simulink model "PassengerCar"  (R2019b)
settings: Solver=ode1  StartTime=0  StopTime=25  FixedStep=1.0000000000000000e-003  RelTol=1e-3
InitFcn:
  | sampleTime = str2double(get_param(bdroot, 'FixedStep'));
undefined symbols (not defined in the file or in its folder): AccPedalPos, BrakePedalPos, BrakeSwitch, DiscIntNeverNeededParam, DYNA4, EngSpd, IgnitionSwitch, InitialGear, InitialSpeed, IntendedEngTrq, LeftIndicator, MainBrakePress, MaxGear, MDL, MinGear, RefAcc, RefLane, RefLatPos, RefPath, RefPathCurv, RefSpd, RefSpdPreview, RefSpdRetrospect, RightIndicator, SteeringWheelAng, SteeringWheelTrq, UserDefinedRefValue, vm_const
libraries: UtilitiesLibrary x31, simulink x18, WheelSystemModules x13, LongitudinalControllerModules x13, LateralControllerModules x7, AnimationBusselectorModules x5, EnvironmentModules x5, BasicEngineControlModules x5, MiscellaneousControlModules x5, Animation3Modules x4, AuxiliariesModules x4, TireModules x4
(part 8 of 39)

== system PassengerCar/VehicleControl/VehicleControlOutput ==
  InitialConditions___UNIQUE_1 : Inport  Description=|
      | <name>InitialConditions</name>
      | <comment></comment>
  LongitudinalControl___UNIQUE_1 : Inport  Description=|  Port=2
      | <name>LongitudinalControl</name>
      | <comment></comment>
  LateralControl___UNIQUE_1 : Inport  Description=|  Port=3
      | <name>LateralControl</name>
      | <comment></comment>
  BrakeHydraulicsControl___UNIQUE_1 : Inport  Description=|  Port=4
      | <name>BrakeHydraulicsControl</name>
      | <comment></comment>
  EngineControl___UNIQUE_1 : Inport  Description=|  Port=5
      | <name>EngineControl</name>
      | <comment></comment>
  SuspensionTestRigControl___UNIQUE_1 : Inport  Description=|  Port=6
      | <name>SuspensionTestRigControl</name>
      | <comment></comment>
  TemperatureControl___UNIQUE_1 : Inport  Description=|  Port=7
      | <name>TemperatureControl</name>
      | <comment></comment>
  UserDefinedControl___UNIQUE_1 : Inport  Description=|  Port=8
      | <name>UserDefinedControl</name>
      | <comment></comment>
  __TDO__VehicleControl : BusCreator  Inputs=8
  VehicleControl___UNIQUE_1 : Outport  Description=|  VectorParamsAs1DForOutWhenUnconnected=off
      | <name>InitialConditions</name>
      | <comment></comment>
  wires:
  __TDO__VehicleControl/1 -> VehicleControl___UNIQUE_1/1  "VehicleControl"
  UserDefinedControl___UNIQUE_1/1 -> __TDO__VehicleControl/8  "UserDefinedControl"
  TemperatureControl___UNIQUE_1/1 -> __TDO__VehicleControl/7  "TemperatureControl"
  SuspensionTestRigControl___UNIQUE_1/1 -> __TDO__VehicleControl/6  "SuspensionTestRigControl"
  EngineControl___UNIQUE_1/1 -> __TDO__VehicleControl/5  "EngineControl"
  BrakeHydraulicsControl___UNIQUE_1/1 -> __TDO__VehicleControl/4  "BrakeHydraulicsControl"
  LateralControl___UNIQUE_1/1 -> __TDO__VehicleControl/3  "LateralControl"
  LongitudinalControl___UNIQUE_1/1 -> __TDO__VehicleControl/2  "LongitudinalControl"
  InitialConditions___UNIQUE_1/1 -> __TDO__VehicleControl/1  "InitialConditions"

== system PassengerCar/ControlUnits/ADAS/ADASOutput ==
  __SRC__ADAS.LongitudinalControlIntervention[0;1] : Constant  Value=0.0  OutDataTypeStr=Inherit: Inherit via back propagation
  __SRC__ADAS.PrioritizedADASControl.LimitsActive[0;1] : Constant  Value=0.0  OutDataTypeStr=Inherit: Inherit via back propagation
  __SRC__ADAS.PrioritizedADASControl.LowerLimitBrakePress[Pa] : Constant  Value=0.0  OutDataTypeStr=Inherit: Inherit via back propagation
  __SRC__ADAS.PrioritizedADASControl.LowerLimitTrq[Nm] : Constant  Value=-vm_const('PAR_NOT_GIVEN')  OutDataTypeStr=Inherit: Inherit via back propagation
  __SRC__ADAS.PrioritizedADASControl.UpperLimitTrq[Nm] : Constant  Value=vm_const('PAR_NOT_GIVEN')  OutDataTypeStr=Inherit: Inherit via back propagation
  __TDO__ADAS : BusCreator  Inputs=2
  __TDO__ADAS.PrioritizedADASControl : BusCreator  Inputs=4
  ADAS___UNIQUE_1 : Outport  Description=|  PortDimensions=[5]  VectorParamsAs1DForOutWhenUnconnected=off
      | <name>PrioritizedADASControl.LimitsActive[0;1]</name>
      | <comment></comment>
  wires:
  __SRC__ADAS.PrioritizedADASControl.LimitsActive[0;1]/1 -> __TDO__ADAS.PrioritizedADASControl/1  "LimitsActive[0;1]"
  __TDO__ADAS.PrioritizedADASControl/1 -> __TDO__ADAS/1  "PrioritizedADASControl"
  __SRC__ADAS.PrioritizedADASControl.UpperLimitTrq[Nm]/1 -> __TDO__ADAS.PrioritizedADASControl/2  "UpperLimitTrq[Nm]"
  __SRC__ADAS.PrioritizedADASControl.LowerLimitTrq[Nm]/1 -> __TDO__ADAS.PrioritizedADASControl/3  "LowerLimitTrq[Nm]"
  __SRC__ADAS.PrioritizedADASControl.LowerLimitBrakePress[Pa]/1 -> __TDO__ADAS.PrioritizedADASControl/4  "LowerLimitBrakePress[Pa]"
  __SRC__ADAS.LongitudinalControlIntervention[0;1]/1 -> __TDO__ADAS/2  "LongitudinalControlIntervention[0;1]"
  __TDO__ADAS/1 -> ADAS___UNIQUE_1/1  "ADAS"

== system PassengerCar/ControlUnits/ADAS/DynaComponentInfo ==

== system PassengerCar/ControlUnits/LCU/DynaComponentInfo ==

== system PassengerCar/ControlUnits/LCU/LCUOutput ==
  VehicleLights___UNIQUE_1 : Inport  Description=|
      | <name>VehicleLights</name>
      | <comment></comment>
  __TDO__LCU : BusCreator  Inputs=1
  LCU___UNIQUE_1 : Outport  Description=|  VectorParamsAs1DForOutWhenUnconnected=off
      | <name>VehicleLights</name>
      | <comment></comment>
  wires:
  VehicleLights___UNIQUE_1/1 -> __TDO__LCU/1  "VehicleLights"
  __TDO__LCU/1 -> LCU___UNIQUE_1/1  "LCU"

== system PassengerCar/ControlUnits/StateSensors/DynaComponentInfo ==

== system PassengerCar/ControlUnits/StateSensors/StateSensorsOutput ==
  IMU___UNIQUE_1 : Inport  Description=|
      | <name>IMU</name>
      | <comment></comment>
  __TDO__StateSensors : BusCreator  Inputs=1
  StateSensors___UNIQUE_1 : Outport  Description=|  VectorParamsAs1DForOutWhenUnconnected=off
      | <name>IMU</name>
      | <comment></comment>
  wires:
  IMU___UNIQUE_1/1 -> __TDO__StateSensors/1  "IMU"
  __TDO__StateSensors/1 -> StateSensors___UNIQUE_1/1  "StateSensors"

== system PassengerCar/ControlUnits/VCU/DynaComponentInfo ==

== system PassengerCar/ControlUnits/VCU/InputFromADAS ==
  fromADAS : Inport  Description=|
      | <name>DriverBrakePedalMode[0;1;2]</name>
      | <comment></comment>
  TDBusSelector : BusSelector  OutputSignals=PrioritizedADASControl
  __TDO__PrioritizedADASControl : BusCreator  Inputs=1
  PrioritizedADASControl___UNIQUE_1 : Outport  Description=|
      | <name>PrioritizedADASControl</name>
      | <comment></comment>
  wires:
  fromADAS/1 -> TDBusSelector/1  "ControlSignals"
  TDBusSelector/1 -> __TDO__PrioritizedADASControl/1  "<PrioritizedADASControl>"
  __TDO__PrioritizedADASControl/1 -> PrioritizedADASControl___UNIQUE_1/1  "PrioritizedADASControl"

== system PassengerCar/ControlUnits/VCU/InputFromCTRL ==
  fromCTRL : Inport
  TDBusSelector : BusSelector  OutputSignals=CTRL.LongitudinalControl.AccPedalPos[0_1],CTRL.LongitudinalControl.BrakePedalPos[0_1],CTRL.LongitudinalControl.DriverInfo.MeanEngMaxTrq[Nm],CTRL.LongitudinalControl.DriverInfo.MeanEngDragTrq[Nm],CTRL.LongitudinalControl.DriverInfo.ThirtyPercentAccPedalEngTrq[Nm]
  __TDD__AccPedalPos[0_1] : Demux  Outputs=[1]
  __TDD__BrakePedalPos[0_1] : Demux  Outputs=1
  __TDD__MeanEngDragTrq[Nm] : Demux  Outputs=[1]
  __TDD__MeanEngMaxTrq[Nm] : Demux  Outputs=[1]
  __TDD__ThirtyPercentAccPedalEngTrq[Nm] : Demux  Outputs=[1]
  AccPedalPos[0_1] : Outport  Description=|  PortDimensions=[1]  VectorParamsAs1DForOutWhenUnconnected=off
      | <name>CTRL.LongitudinalControl.AccPedalPos[0_1]</name>
      | <comment>Accelerator pedal position</comment>
  BrakePedalPos[0_1]___UNIQUE_1 : Outport  Description=|  Port=2  VectorParamsAs1DForOutWhenUnconnected=off
      | <name>CTRL.LongitudinalControl.BrakePedalPos[0_1]</name>
      | <comment></comment>
  MeanEngMaxTrq[Nm]___UNIQUE_1 : Outport  Description=|  Port=3  PortDimensions=[1]  VectorParamsAs1DForOutWhenUnconnected=off
      | <name>CTRL.LongitudinalControl.DriverInfo.MeanEngMaxTrq[Nm]</name>
      | <comment></comment>
  MeanEngDragTrq[Nm]___UNIQUE_1 : Outport  Description=|  Port=4  PortDimensions=[1]  VectorParamsAs1DForOutWhenUnconnected=off
      | <name>CTRL.LongitudinalControl.DriverInfo.MeanEngDragTrq[Nm]</name>
      | <comment></comment>
  ThirtyPercentAccPedalEngTrq[Nm]___UNIQUE_1 : Outport  Description=|  Port=5  PortDimensions=[1]
      | <name>CTRL.LongitudinalControl.DriverInfo.ThirtyPercentAccPedalEngTrq[Nm]</name>
      | <comment></comment>
  wires:
  __TDD__ThirtyPercentAccPedalEngTrq[Nm]/1 -> ThirtyPercentAccPedalEngTrq[Nm]___UNIQUE_1/1  "ThirtyPercentAccPedalEngTrq[Nm]"
  __TDD__MeanEngDragTrq[Nm]/1 -> MeanEngDragTrq[Nm]___UNIQUE_1/1  "MeanEngDragTrq[Nm]"
  __TDD__MeanEngMaxTrq[Nm]/1 -> MeanEngMaxTrq[Nm]___UNIQUE_1/1  "MeanEngMaxTrq[Nm]"
  __TDD__BrakePedalPos[0_1]/1 -> BrakePedalPos[0_1]___UNIQUE_1/1  "BrakePedalPos[0_1]"
  __TDD__AccPedalPos[0_1]/1 -> AccPedalPos[0_1]/1  "AccPedalPos[0_1]"
  TDBusSelector/5 -> __TDD__ThirtyPercentAccPedalEngTrq[Nm]/1  "<ThirtyPercentAccPedalEngTrq[Nm]>"
  TDBusSelector/4 -> __TDD__MeanEngDragTrq[Nm]/1  "<MeanEngDragTrq[Nm]>"
  TDBusSelector/3 -> __TDD__MeanEngMaxTrq[Nm]/1  "<MeanEngMaxTrq[Nm]>"
  TDBusSelector/2 -> __TDD__BrakePedalPos[0_1]/1  "<BrakePedalPos[0_1]>"
  TDBusSelector/1 -> __TDD__AccPedalPos[0_1]/1  "<AccPedalPos[0_1]>"
  fromCTRL/1 -> TDBusSelector/1

== system PassengerCar/ControlUnits/VCU/InputFromVehicle ==
  fromVehicle : Inport
  TDBusSelector : BusSelector  OutputSignals=BrakeSystem.BrakeSystemPhysics.MaxMainBrakePress[Pa]
  __TDD__MaxMainBrakePress[Pa] : Demux  Outputs=[1]
  MaxMainBrakePress[Pa]___UNIQUE_1 : Outport  Description=|  PortDimensions=[1]  VectorParamsAs1DForOutWhenUnconnected=off
      | <name>BrakeSystem.BrakeSystemPhysics.MaxMainBrakePress[Pa]</name>
      | <comment>Maximum main brake pressure</comment>
  wires:
  fromVehicle/1 -> TDBusSelector/1
  TDBusSelector/1 -> __TDD__MaxMainBrakePress[Pa]/1  "<MaxMainBrakePress[Pa]>"
  __TDD__MaxMainBrakePress[Pa]/1 -> MaxMainBrakePress[Pa]___UNIQUE_1/1  "MaxMainBrakePress[Pa]"

== system PassengerCar/ControlUnits/VCU/VCUOutput ==
  TransmissionLoad[0_1]___UNIQUE_1 : Inport  Description=|  PortDimensions=[1]
      | <name>TransmissionLoad[0_1]</name>
      | <comment></comment>
  IntendedEngTrq[Nm]___UNIQUE_1 : Inport  Description=|  Port=2  PortDimensions=[1]
      | <name>IntendedEngTrq[Nm]</name>
      | <comment>Intended torque of engine</comment>
  IntendedEngTrqActive[0;1]___UNIQUE_1 : Inport  Description=|  Port=3  PortDimensions=[1]
      | <name>IntendedEngTrqActive[0;1]</name>
      | <comment></comment>
  IntendedMainBrakePress[Pa]___UNIQUE_1 : Inport  Description=|  Port=4  PortDimensions=[1]
      | <name>IntendedMainBrakePress[Pa]</name>
      | <comment></comment>
  IntendedMainBrakePressActive[0;1]___UNIQUE_1 : Inport  Description=|  Port=5  PortDimensions=[1]
      | <name>IntendedMainBrakePressActive[0;1]</name>
      | <comment></comment>
  __SAT__VCU.EngRunPermission[0;1] : Saturate  UpperLimit=1  LowerLimit=0
  __SRC__VCU.DriverInfo.ConventionalVehicleSwitch[0;1] : Constant  Value=1.0  OutDataTypeStr=Inherit: Inherit via back propagation
  __SRC__VCU.DrivingState[-] : Constant  Value=0.0  OutDataTypeStr=Inherit: Inherit via back propagation
  __SRC__VCU.EngRunPermission[0;1] : Constant  Value=1.0  OutDataTypeStr=Inherit: Inherit via back propagation
  __TDD__VCU.IntendedEngTrqActive[0;1] : Demux  Outputs=[1]
  __TDD__VCU.IntendedEngTrq[Nm] : Demux  Outputs=[1]
  __TDD__VCU.IntendedMainBrakePressActive[0;1] : Demux  Outputs=[1]
  __TDD__VCU.IntendedMainBrakePress[Pa] : Demux  Outputs=[1]
  __TDD__VCU.TransmissionLoad[0_1] : Demux  Outputs=[1]
  __TDO__VCU : BusCreator  Inputs=8
  __TDO__VCU.DriverInfo : BusCreator  Inputs=1
  VCU___UNIQUE_1 : Outport  Description=|  PortDimensions=[8]  VectorParamsAs1DForOutWhenUnconnected=off
      | <name>TransmissionLoad[0_1]</name>
      | <comment></comment>
  wires:
  __SRC__VCU.EngRunPermission[0;1]/1 -> __SAT__VCU.EngRunPermission[0;1]/1
  TransmissionLoad[0_1]___UNIQUE_1/1 -> __TDD__VCU.TransmissionLoad[0_1]/1
  __TDD__VCU.TransmissionLoad[0_1]/1 -> __TDO__VCU/1  "TransmissionLoad[0_1]"
  IntendedEngTrq[Nm]___UNIQUE_1/1 -> __TDD__VCU.IntendedEngTrq[Nm]/1
  __TDD__VCU.IntendedEngTrq[Nm]/1 -> __TDO__VCU/2  "IntendedEngTrq[Nm]"
  IntendedEngTrqActive[0;1]___UNIQUE_1/1 -> __TDD__VCU.IntendedEngTrqActive[0;1]/1
  __TDD__VCU.IntendedEngTrqActive[0;1]/1 -> __TDO__VCU/3  "IntendedEngTrqActive[0;1]"
  IntendedMainBrakePress[Pa]___UNIQUE_1/1 -> __TDD__VCU.IntendedMainBrakePress[Pa]/1
  __TDD__VCU.IntendedMainBrakePress[Pa]/1 -> __TDO__VCU/4  "IntendedMainBrakePress[Pa]"
  IntendedMainBrakePressActive[0;1]___UNIQUE_1/1 -> __TDD__VCU.IntendedMainBrakePressActive[0;1]/1
  __TDD__VCU.IntendedMainBrakePressActive[0;1]/1 -> __TDO__VCU/5  "IntendedMainBrakePressActive[0;1]"
  __SRC__VCU.DrivingState[-]/1 -> __TDO__VCU/6  "DrivingState[-]"
  __SRC__VCU.DriverInfo.ConventionalVehicleSwitch[0;1]/1 -> __TDO__VCU.DriverInfo/1  "ConventionalVehicleSwitch[0;1]"
  __TDO__VCU.DriverInfo/1 -> __TDO__VCU/7  "DriverInfo"
  __SAT__VCU.EngRunPermission[0;1]/1 -> __TDO__VCU/8  "EngRunPermission[0;1]"
  __TDO__VCU/1 -> VCU___UNIQUE_1/1  "VCU"

== system PassengerCar/Environment/Road/DynaSystemInfo ==

== system PassengerCar/Traffic/TrafficOutputs/DistanceToVehicleOutput ==
  LeftAdjacentLaneFrontalDist[m]___UNIQUE_1 : Inport  Description=|  PortDimensions=[1]
      | <name>LeftAdjacentLaneFrontalDist[m]</name>
      | <comment>Distance of VuT to next frontal traffic object on left adjacent lane</comment>
  LeftAdjacentLaneRearDist[m]___UNIQUE_1 : Inport  Description=|  Port=2  PortDimensions=[1]
      | <name>LeftAdjacentLaneRearDist[m]</name>
      | <comment>Distance of VuT to next rear traffic object on left adjacent lane</comment>
  MyLaneFrontalDist[m]___UNIQUE_1 : Inport  Description=|  Port=3  PortDimensions=[1]
      | <name>MyLaneFrontalDist[m]</name>
      | <comment>Distance of VuT to next frontal traffic object on the same lane</comment>
  MyLaneRearDist[m]___UNIQUE_1 : Inport  Description=|  Port=4  PortDimensions=[1]
      | <name>MyLaneRearDist[m]</name>
      | <comment>Distance of VuT to next rear traffic object on the same lane</comment>
  RightAdjacentLaneFrontalDist[m]___UNIQUE_1 : Inport  Description=|  Port=5  PortDimensions=[1]
      | <name>RightAdjacentLaneFrontalDist[m]</name>
      | <comment>Distance of VuT to next frontal traffic object on right adjacent lane</comment>
  RightAdjacentLaneRearDist[m]___UNIQUE_1 : Inport  Description=|  Port=6  PortDimensions=[1]
      | <name>RightAdjacentLaneRearDist[m]</name>
      | <comment>Distance of VuT to next rear traffic object on right adjacent lane</comment>
  LeftAdjacentLaneFrontalSpd[m/s]___UNIQUE_1 : Inport  Description=|  Port=7  PortDimensions=[1]
      | <name>LeftAdjacentLaneFrontalSpd[m/s]</name>
      | <comment>Longitudinal speed of next frontal traffic object on left adjacent lane</comment>
  LeftAdjacentLaneRearSpd[m/s]___UNIQUE_1 : Inport  Description=|  Port=8  PortDimensions=[1]
      | <name>LeftAdjacentLaneRearSpd[m/s]</name>
      | <comment>Longitudinal speed of next rear traffic object on left adjacent lane</comment>
  MyLaneFrontalSpd[m/s]___UNIQUE_1 : Inport  Description=|  Port=9  PortDimensions=[1]
      | <name>MyLaneFrontalSpd[m/s]</name>
      | <comment>Longitudinal speed of next frontal traffic object on the same lane</comment>
  MyLaneRearSpd[m/s]___UNIQUE_1 : Inport  Description=|  Port=10  PortDimensions=[1]
      | <name>MyLaneRearSpd[m/s]</name>
      | <comment>Longitudinal speed of next rear traffic object on the same lane</comment>
  RightAdjacentLaneFrontalSpd[m/s]___UNIQUE_1 : Inport  Description=|  Port=11  PortDimensions=[1]
      | <name>RightAdjacentLaneFrontalSpd[m/s]</name>
      | <comment>Longitudinal speed of next frontal traffic object on right adjacent lane</comment>
  RightAdjacentLaneRearSpd[m/s]___UNIQUE_1 : Inport  Description=|  Port=12  PortDimensions=[1]
      | <name>RightAdjacentLaneRearSpd[m/s]</name>
      | <comment>Longitudinal speed of next rear traffic object on right adjacent lane</comment>
  __TDD__Traffic.AdjacentObjectsSpeeds.LeftAdjacentLaneFrontalSpd[m/s] : Demux  Outputs=[1]
  __TDD__Traffic.AdjacentObjectsSpeeds.LeftAdjacentLaneRearSpd[m/s] : Demux  Outputs=[1]
  __TDD__Traffic.AdjacentObjectsSpeeds.MyLaneFrontalSpd[m/s] : Demux  Outputs=[1]
  __TDD__Traffic.AdjacentObjectsSpeeds.MyLaneRearSpd[m/s] : Demux  Outputs=[1]
  __TDD__Traffic.AdjacentObjectsSpeeds.RightAdjacentLaneFrontalSpd[m/s] : Demux  Outputs=[1]
  __TDD__Traffic.AdjacentObjectsSpeeds.RightAdjacentLaneRearSpd[m/s] : Demux  Outputs=[1]
  __TDD__Traffic.DistancesToVehicle.LeftAdjacentLaneFrontalDist[m] : Demux  Outputs=[1]
  __TDD__Traffic.DistancesToVehicle.LeftAdjacentLaneRearDist[m] : Demux  Outputs=[1]
  __TDD__Traffic.DistancesToVehicle.MyLaneFrontalDist[m] : Demux  Outputs=[1]
  __TDD__Traffic.DistancesToVehicle.MyLaneRearDist[m] : Demux  Outputs=[1]
  __TDD__Traffic.DistancesToVehicle.RightAdjacentLaneFrontalDist[m] : Demux  Outputs=[1]
  __TDD__Traffic.DistancesToVehicle.RightAdjacentLaneRearDist[m] : Demux  Outputs=[1]
  __TDO__Traffic : BusCreator  Inputs=2
  __TDO__Traffic.AdjacentObjectsSpeeds : BusCreator  Inputs=6
  __TDO__Traffic.DistancesToVehicle : BusCreator  Inputs=6
  Traffic___UNIQUE_1 : Outport  Description=|  PortDimensions=[12]  VectorParamsAs1DForOutWhenUnconnected=off
      | <name>LeftAdjacentLaneFrontalDist[m]</name>
      | <comment>Distance of VuT to next frontal traffic object on left adjacent lane</comment>
  wires:
  LeftAdjacentLaneFrontalDist[m]___UNIQUE_1/1 -> __TDD__Traffic.DistancesToVehicle.LeftAdjacentLaneFrontalDist[m]/1
  __TDD__Traffic.DistancesToVehicle.LeftAdjacentLaneFrontalDist[m]/1 -> __TDO__Traffic.DistancesToVehicle/1  "LeftAdjacentLaneFrontalDist[m]"
  __TDO__Traffic.DistancesToVehicle/1 -> __TDO__Traffic/1  "DistancesToVehicle"
  LeftAdjacentLaneRearDist[m]___UNIQUE_1/1 -> __TDD__Traffic.DistancesToVehicle.LeftAdjacentLaneRearDist[m]/1
  __TDD__Traffic.DistancesToVehicle.LeftAdjacentLaneRearDist[m]/1 -> __TDO__Traffic.DistancesToVehicle/2  "LeftAdjacentLaneRearDist[m]"
  MyLaneFrontalDist[m]___UNIQUE_1/1 -> __TDD__Traffic.DistancesToVehicle.MyLaneFrontalDist[m]/1
  __TDD__Traffic.DistancesToVehicle.MyLaneFrontalDist[m]/1 -> __TDO__Traffic.DistancesToVehicle/3  "MyLaneFrontalDist[m]"
  MyLaneRearDist[m]___UNIQUE_1/1 -> __TDD__Traffic.DistancesToVehicle.MyLaneRearDist[m]/1
  __TDD__Traffic.DistancesToVehicle.MyLaneRearDist[m]/1 -> __TDO__Traffic.DistancesToVehicle/4  "MyLaneRearDist[m]"
  RightAdjacentLaneFrontalDist[m]___UNIQUE_1/1 -> __TDD__Traffic.DistancesToVehicle.RightAdjacentLaneFrontalDist[m]/1
  __TDD__Traffic.DistancesToVehicle.RightAdjacentLaneFrontalDist[m]/1 -> __TDO__Traffic.DistancesToVehicle/5  "RightAdjacentLaneFrontalDist[m]"
  RightAdjacentLaneRearDist[m]___UNIQUE_1/1 -> __TDD__Traffic.DistancesToVehicle.RightAdjacentLaneRearDist[m]/1
  __TDD__Traffic.DistancesToVehicle.RightAdjacentLaneRearDist[m]/1 -> __TDO__Traffic.DistancesToVehicle/6  "RightAdjacentLaneRearDist[m]"
  LeftAdjacentLaneFrontalSpd[m/s]___UNIQUE_1/1 -> __TDD__Traffic.AdjacentObjectsSpeeds.LeftAdjacentLaneFrontalSpd[m/s]/1
  __TDD__Traffic.AdjacentObjectsSpeeds.LeftAdjacentLaneFrontalSpd[m/s]/1 -> __TDO__Traffic.AdjacentObjectsSpeeds/1  "LeftAdjacentLaneFrontalSpd[m/s]"
  __TDO__Traffic.AdjacentObjectsSpeeds/1 -> __TDO__Traffic/2  "AdjacentObjectsSpeeds"
  LeftAdjacentLaneRearSpd[m/s]___UNIQUE_1/1 -> __TDD__Traffic.AdjacentObjectsSpeeds.LeftAdjacentLaneRearSpd[m/s]/1
  __TDD__Traffic.AdjacentObjectsSpeeds.LeftAdjacentLaneRearSpd[m/s]/1 -> __TDO__Traffic.AdjacentObjectsSpeeds/2  "LeftAdjacentLaneRearSpd[m/s]"
  MyLaneFrontalSpd[m/s]___UNIQUE_1/1 -> __TDD__Traffic.AdjacentObjectsSpeeds.MyLaneFrontalSpd[m/s]/1
  __TDD__Traffic.AdjacentObjectsSpeeds.MyLaneFrontalSpd[m/s]/1 -> __TDO__Traffic.AdjacentObjectsSpeeds/3  "MyLaneFrontalSpd[m/s]"
  MyLaneRearSpd[m/s]___UNIQUE_1/1 -> __TDD__Traffic.AdjacentObjectsSpeeds.MyLaneRearSpd[m/s]/1
  __TDD__Traffic.AdjacentObjectsSpeeds.MyLaneRearSpd[m/s]/1 -> __TDO__Traffic.AdjacentObjectsSpeeds/4  "MyLaneRearSpd[m/s]"
  RightAdjacentLaneFrontalSpd[m/s]___UNIQUE_1/1 -> __TDD__Traffic.AdjacentObjectsSpeeds.RightAdjacentLaneFrontalSpd[m/s]/1
  __TDD__Traffic.AdjacentObjectsSpeeds.RightAdjacentLaneFrontalSpd[m/s]/1 -> __TDO__Traffic.AdjacentObjectsSpeeds/5  "RightAdjacentLaneFrontalSpd[m/s]"
  RightAdjacentLaneRearSpd[m/s]___UNIQUE_1/1 -> __TDD__Traffic.AdjacentObjectsSpeeds.RightAdjacentLaneRearSpd[m/s]/1
  __TDD__Traffic.AdjacentObjectsSpeeds.RightAdjacentLaneRearSpd[m/s]/1 -> __TDO__Traffic.AdjacentObjectsSpeeds/6  "RightAdjacentLaneRearSpd[m/s]"
  __TDO__Traffic/1 -> Traffic___UNIQUE_1/1  "Traffic"

== system PassengerCar/Vehicle/Auxiliaries/AuxiliariesOutput ==
  GeneratorCurr[A]___UNIQUE_1 : Inport  Description=|  PortDimensions=[1]
      | <name>GeneratorCurr[A]</name>
      | <comment></comment>
  GeneratorTrq[Nm]___UNIQUE_1 : Inport  Description=|  Port=2  PortDimensions=[1]
      | <name>GeneratorTrq[Nm]</name>
      | <comment></comment>
  GeneratorInrt[kgm^2]___UNIQUE_1 : Inport  Description=|  Port=3  PortDimensions=[1]
      | <name>GeneratorInrt[kgm^2]</name>
      | <comment></comment>
  StarterCurr[A]___UNIQUE_1 : Inport  Description=|  Port=4  PortDimensions=[1]
      | <name>StarterCurr[A]</name>
      | <comment></comment>
  StarterTrq[Nm]___UNIQUE_1 : Inport  Description=|  Port=5  PortDimensions=[1]
      | <name>StarterTrq[Nm]</name>
      | <comment></comment>
  StarterInrt[kgm**2]___UNIQUE_1 : Inport  Description=|  Port=6  PortDimensions=[1]
      | <name>StarterInrt[kgm**2]</name>
      | <comment></comment>
  __TDD__Auxiliaries.GeneratorCurr[A] : Demux  Outputs=[1]
  __TDD__Auxiliaries.GeneratorInrt[kgm^2] : Demux  Outputs=[1]
  __TDD__Auxiliaries.GeneratorTrq[Nm] : Demux  Outputs=[1]
  __TDD__Auxiliaries.StarterCurr[A] : Demux  Outputs=[1]
  __TDD__Auxiliaries.StarterInrt[kgm**2] : Demux  Outputs=[1]
  __TDD__Auxiliaries.StarterTrq[Nm] : Demux  Outputs=[1]
  __TDO__Auxiliaries : BusCreator  Inputs=6
  Auxiliaries___UNIQUE_1 : Outport  Description=|  PortDimensions=[6]  VectorParamsAs1DForOutWhenUnconnected=off
      | <name>GeneratorCurr[A]</name>
      | <comment></comment>
  wires:
  __TDO__Auxiliaries/1 -> Auxiliaries___UNIQUE_1/1  "Auxiliaries"
  __TDD__Auxiliaries.StarterInrt[kgm**2]/1 -> __TDO__Auxiliaries/6  "StarterInrt[kgm**2]"
  StarterInrt[kgm**2]___UNIQUE_1/1 -> __TDD__Auxiliaries.StarterInrt[kgm**2]/1
  __TDD__Auxiliaries.StarterTrq[Nm]/1 -> __TDO__Auxiliaries/5  "StarterTrq[Nm]"
  StarterTrq[Nm]___UNIQUE_1/1 -> __TDD__Auxiliaries.StarterTrq[Nm]/1
  __TDD__Auxiliaries.StarterCurr[A]/1 -> __TDO__Auxiliaries/4  "StarterCurr[A]"
  StarterCurr[A]___UNIQUE_1/1 -> __TDD__Auxiliaries.StarterCurr[A]/1
  __TDD__Auxiliaries.GeneratorInrt[kgm^2]/1 -> __TDO__Auxiliaries/3  "GeneratorInrt[kgm^2]"
  GeneratorInrt[kgm^2]___UNIQUE_1/1 -> __TDD__Auxiliaries.GeneratorInrt[kgm^2]/1
  __TDD__Auxiliaries.GeneratorTrq[Nm]/1 -> __TDO__Auxiliaries/2  "GeneratorTrq[Nm]"
  GeneratorTrq[Nm]___UNIQUE_1/1 -> __TDD__Auxiliaries.GeneratorTrq[Nm]/1
  __TDD__Auxiliaries.GeneratorCurr[A]/1 -> __TDO__Auxiliaries/1  "GeneratorCurr[A]"
  GeneratorCurr[A]___UNIQUE_1/1 -> __TDD__Auxiliaries.GeneratorCurr[A]/1

== system PassengerCar/Vehicle/Auxiliaries/DynaComponentInfo ==

== system PassengerCar/Vehicle/Auxiliaries/Generator ==
  EngSpd [rad/s] : Inport
  GeneratorVoltage [V] : Inport  Port=2
  RefVoltage [V] : Inport  Port=3
  LRTime [s] : Inport  Port=4
  Temp [K] : Inport  Port=5
  BattVoltage [V] : Inport  Port=6
  Alternator : AuxiliariesModules/Alternator  DATA_NODE=MDL.Vehicle.Auxiliaries.Alternator  trq_table=MDL.Vehicle.Auxiliaries.Alternator.TrqMap  max_current=MDL.Vehicle.Auxiliaries.Alternator.MaxCurrMap  max_current_rate=MDL.Vehicle.Auxiliaries.Alternator.MaxCurrRate  ref_volt=MDL.Vehicle.Auxiliaries.Alternator.RefVoltage  resist=MDL.Vehicle.Auxiliaries.Alternator.Resist  ratio=MDL.Vehicle.Auxiliaries.Alternator.SpdRatio  Inrt=MDL.Vehicle.Auxiliaries.Alternator.Inrt
  InitCurr [A] : Constant  Value=0
  VoltageRegulator : AuxiliariesModules/VoltageRegulator  DATA_NODE=MDL.Vehicle.Auxiliaries.VoltageRegulator  min_lr=MDL.Vehicle.Auxiliaries.VoltageRegulator.MinLoadResponseTime  LR_thres=MDL.Vehicle.Auxiliaries.VoltageRegulator.LoadResponseSpdLimit
  Curr [A] : Outport  VectorParamsAs1DForOutWhenUnconnected=off
  Trq [Nm] : Outport  Port=2  VectorParamsAs1DForOutWhenUnconnected=off
  Inrt [kgm**2] : Outport  Port=3  VectorParamsAs1DForOutWhenUnconnected=off
  wires:
  VoltageRegulator/1 -> Alternator/1
  EngSpd [rad/s]/1 -> VoltageRegulator/1, Alternator/2
  GeneratorVoltage [V]/1 -> Alternator/3
  InitCurr [A]/1 -> VoltageRegulator/5
  Alternator/4 -> VoltageRegulator/6
  RefVoltage [V]/1 -> VoltageRegulator/3
  LRTime [s]/1 -> VoltageRegulator/4
  Alternator/1 -> Curr [A]/1
  Alternator/2 -> Trq [Nm]/1
  Alternator/3 -> Inrt [kgm**2]/1
  Temp [K]/1 -> Alternator/4
  BattVoltage [V]/1 -> VoltageRegulator/2

== system PassengerCar/Vehicle/Auxiliaries/InputFromCTRL ==
  fromCTRL : Inport
  TDBusSelector : BusSelector  OutputSignals=CTRL.LongitudinalControl.StarterSwitch[0;1],CTRL.EnvironmentalConditions.AmbTemp[K]
  __TDD__AmbTemp[K] : Demux  Outputs=[1]
  __TDD__StarterSwitch[0;1] : Demux  Outputs=[1]
  StarterSwitch[0;1]___UNIQUE_1 : Outport  Description=|  PortDimensions=[1]  VectorParamsAs1DForOutWhenUnconnected=off
      | <name>CTRL.LongitudinalControl.StarterSwitch[0;1]</name>
      | <comment>Engine starter switch</comment>
  AmbTemp[K]___UNIQUE_1 : Outport  Description=|  Port=2  PortDimensions=[1]  VectorParamsAs1DForOutWhenUnconnected=off
      | <name>CTRL.EnvironmentalConditions.AmbTemp[K]</name>
      | <comment></comment>
  wires:
  __TDD__AmbTemp[K]/1 -> AmbTemp[K]___UNIQUE_1/1  "AmbTemp[K]"
  __TDD__StarterSwitch[0;1]/1 -> StarterSwitch[0;1]___UNIQUE_1/1  "StarterSwitch[0;1]"
  TDBusSelector/2 -> __TDD__AmbTemp[K]/1  "<AmbTemp[K]>"
  TDBusSelector/1 -> __TDD__StarterSwitch[0;1]/1  "<StarterSwitch[0;1]>"
  fromCTRL/1 -> TDBusSelector/1

== system PassengerCar/Vehicle/Auxiliaries/InputFromDrivetrain ==
  fromDrivetrain : Inport
  TDBusSelector : BusSelector  OutputSignals=DrivetrainPhysics.EngSpd[rad/s]
  __TDD__EngSpd[rad/s] : Demux  Outputs=1
  EngSpd[rad/s] : Outport  Description=|  VectorParamsAs1DForOutWhenUnconnected=off
      | <name>DrivetrainPhysics.EngSpd[rad/s]</name>
      | <comment></comment>
  wires:
  __TDD__EngSpd[rad/s]/1 -> EngSpd[rad/s]/1  "EngSpd[rad/s]"
  TDBusSelector/1 -> __TDD__EngSpd[rad/s]/1  "<EngSpd[rad/s]>"
  fromDrivetrain/1 -> TDBusSelector/1

== system PassengerCar/Vehicle/Auxiliaries/InputFromElectricalSystem ==
  fromPowernet : Inport
  TDBusSelector : BusSelector  OutputSignals=GeneratorVoltage[V],LowVoltageBattery.LowVoltageBatteryVoltage[V],StarterVoltage[V]
  __TDD__GeneratorVoltage[V] : Demux  Outputs=[1]
  __TDD__LowVoltageBatteryVoltage[V] : Demux  Outputs=[1]
  __TDD__StarterVoltage[V] : Demux  Outputs=[1]
  GeneratorVoltage[V]___UNIQUE_1 : Outport  Description=|  PortDimensions=[1]  VectorParamsAs1DForOutWhenUnconnected=off
      | <name>GeneratorVoltage[V]</name>
      | <comment></comment>
  LowVoltageBatteryVoltage[V]___UNIQUE_1 : Outport  Description=|  Port=2  PortDimensions=[1]  VectorParamsAs1DForOutWhenUnconnected=off
      | <name>LowVoltageBattery.LowVoltageBatteryVoltage[V]</name>
      | <comment></comment>
  StarterVoltage[V]___UNIQUE_1 : Outport  Description=|  Port=3  PortDimensions=[1]  VectorParamsAs1DForOutWhenUnconnected=off
      | <name>StarterVoltage[V]</name>
      | <comment></comment>
  wires:
  __TDD__StarterVoltage[V]/1 -> StarterVoltage[V]___UNIQUE_1/1  "StarterVoltage[V]"
  __TDD__LowVoltageBatteryVoltage[V]/1 -> LowVoltageBatteryVoltage[V]___UNIQUE_1/1  "LowVoltageBatteryVoltage[V]"
  __TDD__GeneratorVoltage[V]/1 -> GeneratorVoltage[V]___UNIQUE_1/1  "GeneratorVoltage[V]"
  TDBusSelector/3 -> __TDD__StarterVoltage[V]/1  "<StarterVoltage[V]>"
  TDBusSelector/2 -> __TDD__LowVoltageBatteryVoltage[V]/1  "<LowVoltageBatteryVoltage[V]>"
  TDBusSelector/1 -> __TDD__GeneratorVoltage[V]/1  "<GeneratorVoltage[V]>"
  fromPowernet/1 -> TDBusSelector/1

== system PassengerCar/Vehicle/Auxiliaries/SimpleEnergyManagement ==
  StarterSwitch [0;1] : Inport
  Generator off : Constant  Value=0
  GeneratorReferenceVoltage : LookupTableModules/ConstantVoltage  DATA_NODE=MDL.Vehicle.Auxiliaries.GeneratorReferenceVoltage  ConstVoltage=MDL.Vehicle.Auxiliaries.GeneratorReferenceVoltage.Voltage
  Switch : Switch  Threshold=0.5
  RefVoltage [V] : Outport  VectorParamsAs1DForOutWhenUnconnected=off
  wires:
  GeneratorReferenceVoltage/1 -> Switch/3
  Switch/1 -> RefVoltage [V]/1
  StarterSwitch [0;1]/1 -> Switch/2
  Generator off/1 -> Switch/1

== system PassengerCar/Vehicle/Auxiliaries/Starter ==
  StarterVoltage [V] : Inport
  EngSpd [rad/s] : Inport  Port=2
  StarterSwitch [0;1] : Inport  Port=3
  Temp [K] : Inport  Port=4
  PermanentMagnetDCMotor : AuxiliariesModules/PermanentMagnetDCMotor  DATA_NODE=MDL.Vehicle.Auxiliaries.PermanentMagnetDCMotor  flux=MDL.Vehicle.Auxiliaries.PermanentMagnetDCMotor.FieldFlux  armature_inductance=MDL.Vehicle.Auxiliaries.PermanentMagnetDCMotor.ArmatureInduct  armature_resistance=MDL.Vehicle.Auxiliaries.PermanentMagnetDCMotor.ArmatureResistCurve  motor_const=MDL.Vehicle.Auxiliaries.PermanentMagnetDCMotor.MotorConst  inrt=MDL.Vehicle.Auxiliaries.PermanentMagnetDCMotor.Inrt  heat_cap=MDL.Vehicle.Auxiliaries.PermanentMagnetDCMotor.HeatCap
  StarterControl : AuxiliariesModules/StarterControl  DATA_NODE=MDL.Vehicle.Auxiliaries.StarterControl  speedratio=MDL.Vehicle.Auxiliaries.StarterControl.StarterEngSpdRatio
  Terminator : Terminator
  Terminator1 : Terminator
  Terminator2 : Terminator
  StarterCurr [A] : Outport  VectorParamsAs1DForOutWhenUnconnected=off
  StarterTrq [Nm] : Outport  Port=2  VectorParamsAs1DForOutWhenUnconnected=off
  StarterInrt [kgm**2] : Outport  Port=3  VectorParamsAs1DForOutWhenUnconnected=off
  wires:
  PermanentMagnetDCMotor/4 -> StarterControl/6
  StarterControl/1 -> StarterCurr [A]/1
  StarterControl/2 -> StarterTrq [Nm]/1
  StarterControl/3 -> StarterInrt [kgm**2]/1
  StarterControl/4 -> PermanentMagnetDCMotor/1
  StarterControl/5 -> PermanentMagnetDCMotor/3
  PermanentMagnetDCMotor/1 -> StarterControl/4
  StarterVoltage [V]/1 -> StarterControl/1
  EngSpd [rad/s]/1 -> StarterControl/3
  StarterSwitch [0;1]/1 -> StarterControl/2
  PermanentMagnetDCMotor/3 -> StarterControl/5
  Temp [K]/1 -> PermanentMagnetDCMotor/2
  PermanentMagnetDCMotor/2 -> Terminator/1
  PermanentMagnetDCMotor/5 -> Terminator1/1
  PermanentMagnetDCMotor/6 -> Terminator2/1

== system PassengerCar/Vehicle/BrakeSystem/BrakeSystemControlUnit ==
  fromBrakeSystemPhysics : Inport
  fromCTRL : Inport  Port=2
  fromWheelSystem : Inport  Port=3
  fromChassis : Inport  Port=4
  BasicElectronicStabilityControl : Subsystem
  BasicElectronicStabilityControlInput : Subsystem
  BrakeSystemControlUnitOutput : Subsystem  Tag=TESIS DYNAware Interface Block  mask{NeedsUpdate=off, SignalInfo=|}
      mask SignalInfo=|
      | {
      |   "Version": "4.6",
      |   "MuxedOutputBusName": "BrakeSystemControlUnit",
      |   "MuxedInputBusName": "input",
      |   "MuxedInputSelected": false,
      |   "MuxedOutputSelected": true,
      |   "SignalData": [
      |     {
      |       "initialValue": "0.0",
      |       "name": "FrontLeftWheelBrakePress[Pa]",
      |       "comment": "Front left wheel brake pressure",
      |       "minString": "",
      |       "maxString": "",
      |       "width": 1,
      |       "dataType": 0,
      |       "signalType": 0,
      |       "createSignal": false,
      |       "outputName": "FrontLeftWheelBrakePress[Pa]",
      |       "generateSignalAccessBlock": false,
      |       "accessId": "$(parentId).$(blockName).$(outputName)"
      |     },
      |     {
      |       "initialValue": "0.0",
      |       "name": "FrontRightWheelBrakePress[Pa]",
      |       "comment": "Front right wheel brake pressure",
      |       "minString": "",
      |       "maxString": "",
      |       "width": 1,
      |       "dataType": 0,
      |       "signalType": 0,
      |       "createSignal": false,
      |       "outputName": "FrontRightWheelBrakePress[Pa]",
      |       "generateSignalAccessBlock": false,
      |       "accessId": "$(parentId).$(blockName).$(outputName)"
      |     },
      |     {
      |       "initialValue": "0.0",
      |       "name": "RearLeftWheelBrakePress[Pa]",
      |       "comment": "Rear left wheel brake pressure",
      |       "minString": "",
      |       "maxString": "",
      |       "width": 1,
      |       "dataType": 0,
      |       "signalType": 0,
      |       "createSignal": false,
      |       "outputName": "RearLeftWheelBrakePress[Pa]",
      |       "generateSignalAccessBlock": false,
      |       "accessId": "$(parentId).$(blockName).$(outputName)"
      |     },
      |     {
      |       "initialValue": "0.0",
      |       "name": "RearRightWheelBrakePress[Pa]",
      |       "comment": "Rear right wheel brake pressure",
      |       "minString": "",
      |       "maxString": "",
      |       "width": 1,
      |       "dataType": 0,
      |       "signalType": 0,
      |       "createSignal": false,
      |       "outputName": "RearRightWheelBrakePress[Pa]",
      |       "generateSignalAccessBlock": false,
      |       "accessId": "$(parentId).$(blockName).$(outputName)"
      |     },
      |     {
      |       "initialValue": "",
      |       "name": "Rear2LeftWheelBrakePress[Pa]",
      |       "comment": "",
      |       "minString": "",
      |       "maxString": "",
      |       "width": 1,
      |       "dataType": 0,
      |       "signalType": 0,
      |       "createSignal": false,
      |       "outputName": "Rear2LeftWheelBrakePress[Pa]",
      |       "generateSignalAccessBlock": false,
      |       "accessId": "$(parentId).$(blockName).$(outputName)"
      |     },
      |     {
      |       "initialValue": "",
      |       "name": "Rear2RightWheelBrakePress[Pa]",
      |       "comment": "",
      |       "minString": "",
      |       "maxString": "",
      |       "width": 1,
      |       "dataType": 0,
      |       "signalType": 0,
      |       "createSignal": false,
      |       "outputName": "Rear2RightWheelBrakePress[Pa]",
      |       "generateSignalAccessBlock": false,
      |       "accessId": "$(parentId).$(blockName).$(outputName)"
      |     },
      |     {
      |       "initialValue": "",
      |       "name": "Rear3LeftWheelBrakePress[Pa]",
      |       "comment": "",
      |       "minString": "",
      |       "maxString": "",
      |       "width": 1,
      |       "dataType": 0,
      |       "signalType": 0,
      |       "createSignal": false,
      |       "outputName": "Rear3LeftWheelBrakePress[Pa]",
      |       "generateSignalAccessBlock": false,
      |       "accessId": "$(parentId).$(blockName).$(outputName)"
      |     },
      |     {
      |       "initialValue": "",
      |       "name": "Rear3RightWheelBrakePress[Pa]",
      |       "comment": "",
      |       "minString": "",
      |       "maxString": "",
      |       "width": 1,
      |       "dataType": 0,
      |       "signalType": 0,
      |       "createSignal": false,
      |       "outputName": "Rear3RightWheelBrakePress[Pa]",
      |       "generateSignalAccessBlock": false,
      |       "accessId": "$(parentId).$(blockName).$(outputName)"
      |     },
      |     {
      |       "initialValue": "0.0",
      |       "name": "WheelBrakePressActive[0;1]",
      |       "comment": "",
      |       "minString": "",
      |       "maxString": "",
      |       "width": 1,
      |       "dataType": 0,
      |       "signalType": 0,
      |       "createSignal": false,
      |       "outputName": "WheelBrakePressActive[0;1]",
      |       "generateSignalAccessBlock": false,
      |       "accessId": "$(parentId).$(blockName).$(outputName)"
      |     },
      |     {
      |       "initialValue": "0.0",
      |       "name": "ControlUnit.YawStabilityControl",
      |       "comment": "",
      |       "minString": "",
      |       "maxString": "",
      |       "width": -1,
      |       "dataType": 0,
      |       "signalType": 1,
      |       "createSignal": false,
      |       "outputName": "ControlUnit.YawStabilityControl",
      |       "generateSignalAccessBlock": false,
      |       "accessId": "$(parentId).$(blockName).$(outputName)"
      |     },
      |     {
      |       "initialValue": "0.0",
      |       "name": "ControlUnit.AntiLockBrakeSystem",
      |       "comment": "",
      |       "minString": "",
      |       "maxString": "",
      |       "width": -1,
      |       "dataType": 0,
      |       "signalType": 1,
      |       "createSignal": false,
      |       "outputName": "ControlUnit.AntiLockBrakeSystem",
      |       "generateSignalAccessBlock": false,
      |       "accessId": "$(parentId).$(blockName).$(outputName)"
      |     }
      |   ]
      | }
      mask prompts: NeedsUpdate "Specify, if subsystem content needs to be updated"; SignalInfo "Signal Info (json)"
      mask help: DYNA4 Interface Block Version 4.6
      mask init:
      | blockName = get_param(gcbh, 'Name');
      | parentId = DYNA4.ModelHandling.AccessID.getFromHierarchy(gcbh);
      | TD.InterfaceBlock.ModelCallbacks.GenerateContent(gcb);
      settings: DeleteFcn=TD.InterfaceBlock.ModelCallbacks.CloseGUI( gcbh );  NameChangeFcn=TD.InterfaceBlock.ModelCallbacks.BlockRenamedHandler(gcbh);  OpenFcn=TD.InterfaceBlock.ModelCallbacks.OpenGUI( gcbh );  CloseFcn=TD.InterfaceBlock.ModelCallbacks.CloseGUI( gcbh );
      mask Display:
      | image('InterfaceBlock.png','center');
      | port_label('input',1, 'FrontLeftWheelBrakePress[Pa]');
      | port_label('input',2, 'FrontRightWheelBrakePress[Pa]');
      | port_label('input',3, 'RearLeftWheelBrakePress[Pa]');
      | port_label('input',4, 'RearRightWheelBrakePress[Pa]');
      | port_label('input',5, 'Rear2LeftWheelBrakePress[Pa]');
      | port_label('input',6, 'Rear2RightWheelBrakePress[Pa]');
      | port_label('input',7, 'Rear3LeftWheelBrakePress[Pa]');
      | port_label('input',8, 'Rear3RightWheelBrakePress[Pa]');
      | port_label('input',9, 'WheelBrakePressActive[0;1]');
      | port_label('input',10, 'ControlUnit.YawStabilityControl');
      | port_label('input',11, 'ControlUnit.AntiLockBrakeSystem');
      | port_label('output',1, 'BrakeSystemControlUnit');
  Bus Selector : BusSelector  OutputSignals=Active[0;1]
  Bus Selector1 : BusSelector  OutputSignals=Active[0;1]
  Bus Selector2 : BusSelector  OutputSignals=Rear2LeftWheelBrakePress[Pa],Rear2RightWheelBrakePress[Pa],Rear3LeftWheelBrakePress[Pa],Rear3RightWheelBrakePress[Pa]
  Data Type Conversion1 : DataTypeConversion  OutDataTypeStr=double
  Demux : Demux
  DynaComponentInfo : Subsystem  Tag=DynaComponentInfo
      mask init:
      | data= get_param(gcb, 'UserData');
      settings: OpenFcn=DYNA4.ModelHandling.Component.ShowEditComponentInformationDialog(gcb);
      mask Display: disp(['Type = ', data.type, '\nGroup = ', data.group, '\nName = ', data.name ])
  Logical Operator : Logic  Operator=OR  AllPortsSameDT=off  OutDataTypeStr=boolean
  fromBrakeSystemPhysics1 : InportShadow
  BrakeSystemControlUnit : Outport  VectorParamsAs1DForOutWhenUnconnected=off
  wires:
  fromChassis/1 -> BasicElectronicStabilityControlInput/4(fromChassis)
  BasicElectronicStabilityControlInput/28(YawInertia[kgm2]) -> BasicElectronicStabilityControl/28(YawInertia[kgm2])
  BasicElectronicStabilityControlInput/29(FrontWheelTrack[m]) -> BasicElectronicStabilityControl/29(FrontWheelTrack[m])
  BasicElectronicStabilityControlInput/24(RearBrakeTrqPressRatio[m**3]) -> BasicElectronicStabilityControl/24(RearBrakeTrqPressRatio[m**3])
  BasicElectronicStabilityControlInput/27(YawRate[rad/s]) -> BasicElectronicStabilityControl/27(YawRate[rad/s])
  BasicElectronicStabilityControlInput/19(RearRightWheelRotAcc[rad/s**2]) -> BasicElectronicStabilityControl/19(RearRightWheelRotAcc[rad/s**2])
  BasicElectronicStabilityControlInput/20(RearRightTireDynamicRadius[m]) -> BasicElectronicStabilityControl/20(RearRightTireDynamicRadius[m])
  BasicElectronicStabilityControlInput/17(RearRightWheelLongSpd(ContactSys)[m/s]) -> BasicElectronicStabilityControl/17(RearRightWheelLongSpd(ContactSys)[m/s])
  BasicElectronicStabilityControlInput/14(RearLeftWheelRotSpd[rad/s]) -> BasicElectronicStabilityControl/14(RearLeftWheelRotSpd[rad/s])
  BasicElectronicStabilityControlInput/16(RearLeftTireDynamicRadius[m]) -> BasicElectronicStabilityControl/16(RearLeftTireDynamicRadius[m])
  BasicElectronicStabilityControlInput/18(RearRightWheelRotSpd[rad/s]) -> BasicElectronicStabilityControl/18(RearRightWheelRotSpd[rad/s])
  BasicElectronicStabilityControlInput/12(FrontRightTireDynamicRadius[m]) -> BasicElectronicStabilityControl/12(FrontRightTireDynamicRadius[m])
  BasicElectronicStabilityControlInput/13(RearLeftWheelLongSpd(ContactSys)[m/s]) -> BasicElectronicStabilityControl/13(RearLeftWheelLongSpd(ContactSys)[m/s])
  BasicElectronicStabilityControlInput/30(RearWheelTrack[m]) -> BasicElectronicStabilityControl/30(RearWheelTrack[m])
  BasicElectronicStabilityControlInput/15(RearLeftWheelRotAcc[rad/s**2]) -> BasicElectronicStabilityControl/15(RearLeftWheelRotAcc[rad/s**2])
  BasicElectronicStabilityControlInput/22(RearLeftTireRadius[m]) -> BasicElectronicStabilityControl/22(RearLeftTireRadius[m])
  BasicElectronicStabilityControlInput/8(FrontLeftTireDynamicRadius[m]) -> BasicElectronicStabilityControl/8(FrontLeftTireDynamicRadius[m])
  BasicElectronicStabilityControlInput/21(FrontLeftTireRadius[m]) -> BasicElectronicStabilityControl/21(FrontLeftTireRadius[m])
  BasicElectronicStabilityControlInput/9(FrontRightWheelLongSpd(ContactSys)[m/s]) -> BasicElectronicStabilityControl/9(FrontRightWheelLongSpd(ContactSys)[m/s])
  BasicElectronicStabilityControlInput/6(FrontLeftWheelRotSpd[rad/s]) -> BasicElectronicStabilityControl/6(FrontLeftWheelRotSpd[rad/s])
  BasicElectronicStabilityControlInput/4(ESCSwitchFromVehicleControl[0;1]) -> BasicElectronicStabilityControl/4(ESCSwitchFromVehicleControl[0;1])
  BasicElectronicStabilityControlInput/11(FrontRightWheelRotAcc[rad/s**2]) -> BasicElectronicStabilityControl/11(FrontRightWheelRotAcc[rad/s**2])
  BasicElectronicStabilityControlInput/2(WheelBrakePressuresFromBrakeHydraulics[Pa]) -> BasicElectronicStabilityControl/2(WheelBrakePressuresFromBrakeHydraulics[Pa]1)
  BasicElectronicStabilityControlInput/7(FrontLeftWheelRotAcc[rad/s**2]) -> BasicElectronicStabilityControl/7(FrontLeftWheelRotAcc[rad/s**2])
  BasicElectronicStabilityControlInput/3(ABSSwitchFromVehicleControl[0;1]) -> BasicElectronicStabilityControl/3(ABSSwitchFromVehicleControl[0;1])
  Bus Selector2/1 -> BrakeSystemControlUnitOutput/5(Rear2LeftWheelBrakePress[Pa]___UNIQUE_1)  "<Rear2LeftWheelBrakePress[Pa]>"
  Bus Selector2/2 -> BrakeSystemControlUnitOutput/6(Rear2RightWheelBrakePress[Pa]___UNIQUE_1)  "<Rear2RightWheelBrakePress[Pa]>"
  BasicElectronicStabilityControlInput/10(FrontRightWheelRotSpd[rad/s]) -> BasicElectronicStabilityControl/10(FrontRightWheelRotSpd[rad/s])
  fromWheelSystem/1 -> BasicElectronicStabilityControlInput/3(fromWheelSystem)
  fromCTRL/1 -> BasicElectronicStabilityControlInput/2(fromCTRL)
  fromBrakeSystemPhysics/1 -> BasicElectronicStabilityControlInput/1(fromBrakePhysics)
  Bus Selector2/4 -> BrakeSystemControlUnitOutput/8(Rear3RightWheelBrakePress[Pa]___UNIQUE_1)  "<Rear3RightWheelBrakePress[Pa]>"
  BasicElectronicStabilityControl/2(YawStabilityControlInfo) -> BrakeSystemControlUnitOutput/10(YawStabilityControl___UNIQUE_1), Bus Selector/1
  BasicElectronicStabilityControl/3(AntiLockBrakeSystemInfo) -> Bus Selector1/1, BrakeSystemControlUnitOutput/11(AntiLockBrakeSystem___UNIQUE_1)
  BasicElectronicStabilityControlInput/26(Acc_wrt_WorldSys(VehSys)[m/**s2]) -> BasicElectronicStabilityControl/26(Acc_wrt_WorldSys(VehSys)[m/**s2])
  BasicElectronicStabilityControlInput/1(MaxMainBrakePress[Pa]) -> BasicElectronicStabilityControl/1(MaxMainBrakePress[Pa])
  BasicElectronicStabilityControl/1(WheelBrakePressures[Pa]) -> Demux/1
  Demux/3 -> BrakeSystemControlUnitOutput/3(RearLeftWheelBrakePress[Pa]___UNIQUE_1)
  BasicElectronicStabilityControlInput/5(FrontLeftWheelLongSpd(ContactSys)[m/s]) -> BasicElectronicStabilityControl/5(FrontLeftWheelLongSpd(ContactSys)[m/s])
  BasicElectronicStabilityControlInput/25(Vel_wrt_WorldSys(VehSys)[m/s]) -> BasicElectronicStabilityControl/25(Vel_wrt_WorldSys(VehSys)[m/s])
  Bus Selector2/3 -> BrakeSystemControlUnitOutput/7(Rear3LeftWheelBrakePress[Pa]___UNIQUE_1)  "<Rear3LeftWheelBrakePress[Pa]>"
  fromBrakeSystemPhysics1/1 -> Bus Selector2/1
  Logical Operator/1 -> Data Type Conversion1/1
  Data Type Conversion1/1 -> BrakeSystemControlUnitOutput/9(WheelBrakePressActive[0;1]___UNIQUE_1)
  Demux/2 -> BrakeSystemControlUnitOutput/2(FrontRightWheelBrakePress[Pa]___UNIQUE_1)
  BrakeSystemControlUnitOutput/1(BrakeSystemControlUnit___UNIQUE_1) -> BrakeSystemControlUnit/1
  BasicElectronicStabilityControlInput/23(FrontBrakeTrqPressRatio[m**3]) -> BasicElectronicStabilityControl/23(FrontBrakeTrqPressRatio[m**3])
  Demux/4 -> BrakeSystemControlUnitOutput/4(RearRightWheelBrakePress[Pa]___UNIQUE_1)
  Demux/1 -> BrakeSystemControlUnitOutput/1(FrontLeftWheelBrakePress[Pa]___UNIQUE_1)
  Bus Selector/1 -> Logical Operator/1  "<Active[0;1]>"
  Bus Selector1/1 -> Logical Operator/2  "<Active[0;1]>"

== system PassengerCar/Vehicle/BrakeSystem/BrakeSystemOutputs ==
  BrakeSystemPhysics___UNIQUE_1 : Inport  Description=|
      | <name>BrakeSystemPhysics</name>
      | <comment></comment>
  BrakeSystemControlUnitInfo___UNIQUE_1 : Inport  Description=|  Port=2
      | <name>BrakeSystemControlUnitInfo</name>
      | <comment></comment>
  __TDO__BrakeSystem : BusCreator  Inputs=2
  BrakeSystem___UNIQUE_1 : Outport  Description=|  VectorParamsAs1DForOutWhenUnconnected=off
      | <name>BrakeSystemPhysics</name>
      | <comment></comment>
  wires:
  BrakeSystemPhysics___UNIQUE_1/1 -> __TDO__BrakeSystem/1  "BrakeSystemPhysics"
  BrakeSystemControlUnitInfo___UNIQUE_1/1 -> __TDO__BrakeSystem/2  "BrakeSystemControlUnitInfo"
  __TDO__BrakeSystem/1 -> BrakeSystem___UNIQUE_1/1  "BrakeSystem"
